simulink model "fuyangfangzhen"  (R2012b)
settings: Solver=ode3  StartTime=0.0  StopTime=20.0  FixedStep=0.005  RelTol=1e-3
settings Model: Creator=Administrator  LastModifiedBy=Administrator
settings DataIOCC: InspectSignalLogs=on

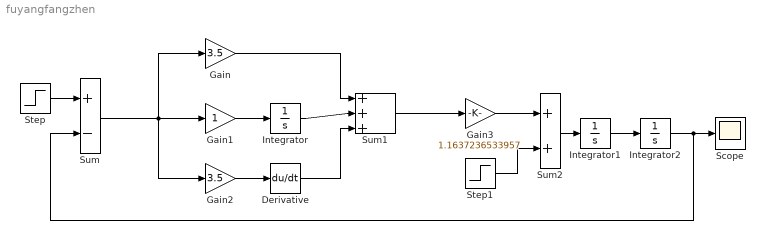
== system fuyangfangzhen ==
  Derivative : Derivative
  Gain : Gain  Gain=3.5
  Gain1 : Gain
  Gain2 : Gain  Gain=3.5
  Gain3 : Gain  Gain=1.1637236533957
  Integrator : Integrator
  Integrator1 : Integrator
  Integrator2 : Integrator
  Scope : Scope
      settings: MaxDataPoints=50000000
  Step : Step  After=0.5  SampleTime=0
  Step1 : Step  Time=2.2577289  SampleTime=0
  Sum : Sum  Inputs=+-
  Sum1 : Sum  Inputs=|+++
  Sum2 : Sum
  wires:
  Step/1 -> Sum/1
  Gain1/1 -> Integrator/1
  Gain2/1 -> Derivative/1
  Sum/1 -> Gain/1, Gain1/1, Gain2/1
  Gain/1 -> Sum1/1
  Integrator/1 -> Sum1/2
  Derivative/1 -> Sum1/3
  Sum1/1 -> Gain3/1
  Gain3/1 -> Sum2/1
  Step1/1 -> Sum2/2
  Sum2/1 -> Integrator1/1
  Integrator1/1 -> Integrator2/1
  Integrator2/1 -> Sum/2, Scope/1
